simulink model "resolver_ekf_validation"  (R2026a)
settings: Solver=FixedStepDiscrete  StopTime=0.2  FixedStep=5e-5
settings Model: Creator=hzldx  LastModifiedBy=hzldx

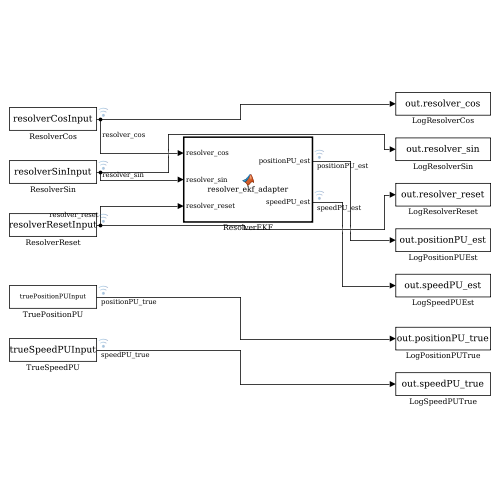
[thumbnail: Simulink's stored preview of the top-level diagram]
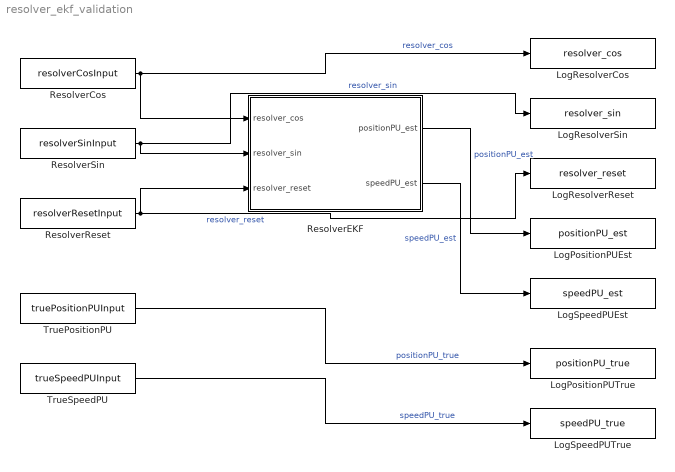
== system resolver_ekf_validation ==
  LogPositionPUEst : ToWorkspace  VariableName=positionPU_est  SaveFormat=Timeseries  SampleTime=-1
  LogPositionPUTrue : ToWorkspace  VariableName=positionPU_true  SaveFormat=Timeseries  SampleTime=-1
  LogResolverCos : ToWorkspace  VariableName=resolver_cos  SaveFormat=Timeseries  SampleTime=-1
  LogResolverReset : ToWorkspace  VariableName=resolver_reset  SaveFormat=Timeseries  SampleTime=-1
  LogResolverSin : ToWorkspace  VariableName=resolver_sin  SaveFormat=Timeseries  SampleTime=-1
  LogSpeedPUEst : ToWorkspace  VariableName=speedPU_est  SaveFormat=Timeseries  SampleTime=-1
  LogSpeedPUTrue : ToWorkspace  VariableName=speedPU_true  SaveFormat=Timeseries  SampleTime=-1
  ResolverCos : FromWorkspace  VariableName=resolverCosInput  SampleTime=5e-5  Interpolate=off  OutputAfterFinalValue=Holding final value
  ResolverEKF : MATLAB Function  TreatAsAtomicUnit=on
  ResolverReset : FromWorkspace  VariableName=resolverResetInput  SampleTime=5e-5  Interpolate=off  OutputAfterFinalValue=Holding final value
  ResolverSin : FromWorkspace  VariableName=resolverSinInput  SampleTime=5e-5  Interpolate=off  OutputAfterFinalValue=Holding final value
  TruePositionPU : FromWorkspace  VariableName=truePositionPUInput  SampleTime=5e-5  Interpolate=off  OutputAfterFinalValue=Holding final value
  TrueSpeedPU : FromWorkspace  VariableName=trueSpeedPUInput  SampleTime=5e-5  Interpolate=off  OutputAfterFinalValue=Holding final value
  wires:
  ResolverCos/1 -> ResolverEKF/1(resolver_cos), LogResolverCos/1  "resolver_cos"
  ResolverSin/1 -> ResolverEKF/2(resolver_sin), LogResolverSin/1  "resolver_sin"
  ResolverReset/1 -> ResolverEKF/3(resolver_reset), LogResolverReset/1  "resolver_reset"
  ResolverEKF/1(positionPU_est) -> LogPositionPUEst/1  "positionPU_est"
  ResolverEKF/2(speedPU_est) -> LogSpeedPUEst/1  "speedPU_est"
  TruePositionPU/1 -> LogPositionPUTrue/1  "positionPU_true"
  TrueSpeedPU/1 -> LogSpeedPUTrue/1  "speedPU_true"

== matlab function resolver_ekf_validation/ResolverEKF ==
  data: resolver_cos input; positionPU_est output; resolver_sin input; resolver_reset input; speedPU_est output; resolver_ekf_config parameter
function [positionPU_est, speedPU_est] = resolver_ekf_adapter(resolver_cos, resolver_sin, resolver_reset, resolver_ekf_config)
%#codegen
persistent state
if isempty(state)
    state = zeros(3, 1);
end
cfg = resolver_ekf_config;
[state, positionPU_est, speedPU_est] = resolver_ekf_step( ...
    state, resolver_cos, resolver_sin, resolver_reset ~= 0, cfg);
end
